simulink model "receive_a429_r2019b"  (R2019b)
settings: Solver=VariableStepAuto  StartTime=0.0  StopTime=10.0  RelTol=1e-3
model workspace (MAT data in the model file):
  ED247Configuration(1).name = 'T11M4_A429_SIMU2SWIM_BUS_1_350_10'
  ED247Configuration(1).direction = 'IN'
  ED247Configuration(1).type = 'uint8'
  ED247Configuration(1).dimensions = 1
  ED247Configuration(1).width = 4
  ED247Configuration(1).size = 4
  ED247Configuration(1).sample_time = 1
  ED247Configuration(1).validity_duration = 1
  ED247Configuration(1).signal_type = 'A429'
  ED247Configuration(1).sample_size = 4
  ED247Configuration(2).name = 'T11M4_A429_SIMU2SWIM_BUS_1_200_10'
  ED247Configuration(2).direction = 'IN'
  ED247Configuration(2).type = 'uint8'
  ED247Configuration(2).dimensions = 1
  ED247Configuration(2).width = 4
  ED247Configuration(2).size = 4
  ED247Configuration(2).sample_time = 1
  ED247Configuration(2).validity_duration = 1
  ED247Configuration(2).signal_type = 'A429'
  ED247Configuration(2).sample_size = 4
  ED247Configuration(3).name = 'T11M4_A429_SIMU2SWIM_BUS_1_200_11'
  ED247Configuration(3).direction = 'IN'
  ED247Configuration(3).type = 'uint8'
  ED247Configuration(3).dimensions = 1
  ED247Configuration(3).width = 4
  ED247Configuration(3).size = 4
  ED247Configuration(3).sample_time = 1
  ED247Configuration(3).validity_duration = 1
  ED247Configuration(3).signal_type = 'A429'
  ED247Configuration(3).sample_size = 4
libraries: lib_ed247 x2
settings Model: EnablePacing=on  Creator=odufour  LastModifiedBy=odufour
settings DebuggingCC: InheritedTsInSrcMsg=none

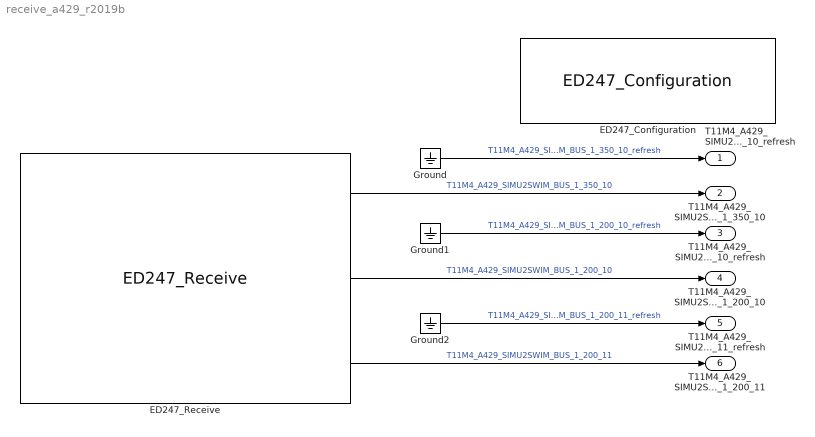
== system receive_a429_r2019b ==
  ED247_Configuration : lib_ed247/ED247_Configuration  configurationFilename='ecic_func_exchange_a429_uc_tester_simple.xml'  enableLog=on  logFilename='<PROJECT_FOLDER>\tests\_files\tmp.log'
      settings: SourceProductName=Airbus ED247
  ED247_Receive : lib_ed247/ED247_Receive  enable_refresh=off  refresh_factor=0  sample_time=-1  show_port_labels=on
      settings: SourceProductName=Airbus ED247
  Ground : Ground
  Ground1 : Ground
  Ground2 : Ground
  T11M4_A429_SIMU2SWIM_BUS_1_350_10_refresh : Outport
  T11M4_A429_SIMU2SWIM_BUS_1_350_10 : Outport  Port=2  OutDataTypeStr=uint8  PortDimensions=4  SampleTime=0.1
  T11M4_A429_SIMU2SWIM_BUS_1_200_10_refresh : Outport  Port=3
  T11M4_A429_SIMU2SWIM_BUS_1_200_10 : Outport  Port=4  OutDataTypeStr=uint8  PortDimensions=4  SampleTime=0.1
  T11M4_A429_SIMU2SWIM_BUS_1_200_11_refresh : Outport  Port=5
  T11M4_A429_SIMU2SWIM_BUS_1_200_11 : Outport  Port=6  OutDataTypeStr=uint8  PortDimensions=4  SampleTime=0.1
  wires:
  Ground/1 -> T11M4_A429_SIMU2SWIM_BUS_1_350_10_refresh/1  "T11M4_A429_SIMU2SWIM_BUS_1_350_10_refresh"
  ED247_Receive/1 -> T11M4_A429_SIMU2SWIM_BUS_1_350_10/1  "T11M4_A429_SIMU2SWIM_BUS_1_350_10"
  Ground1/1 -> T11M4_A429_SIMU2SWIM_BUS_1_200_10_refresh/1  "T11M4_A429_SIMU2SWIM_BUS_1_200_10_refresh"
  ED247_Receive/2 -> T11M4_A429_SIMU2SWIM_BUS_1_200_10/1  "T11M4_A429_SIMU2SWIM_BUS_1_200_10"
  Ground2/1 -> T11M4_A429_SIMU2SWIM_BUS_1_200_11_refresh/1  "T11M4_A429_SIMU2SWIM_BUS_1_200_11_refresh"
  ED247_Receive/3 -> T11M4_A429_SIMU2SWIM_BUS_1_200_11/1  "T11M4_A429_SIMU2SWIM_BUS_1_200_11"
